simulink model "sen_gyro_lib"  (R2020b)
settings: Solver=FixedStepDiscrete  StartTime=0.0  StopTime=20000  FixedStep=sen.imu_rate  RelTol=1e-3
undefined symbols (not defined in the file or in its folder): DiscIntNeverNeededParam, sen, sen_gyro_dyn_zeta, sen_gyro_lpf_wc
libraries: simulink_extras x2
settings Model: Creator=jsint  LastModifiedBy=jsint

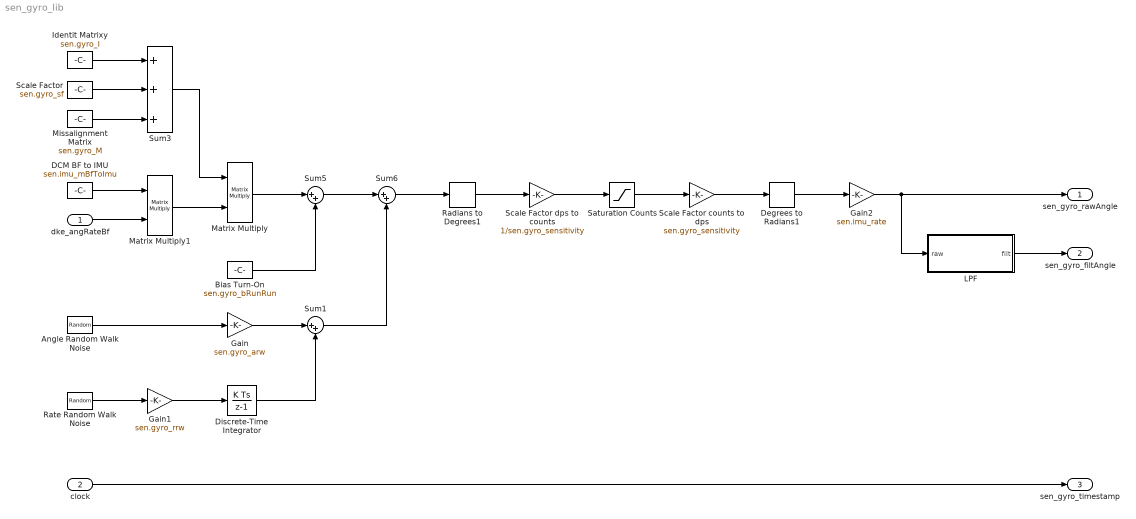
== system sen_gyro_lib ==
  dke_angRateBf : Inport  OutDataTypeStr=double  Unit=rad/s  PortDimensions=[3,1]
  clock : Inport  Port=2  OutDataTypeStr=double  Unit=s  PortDimensions=[1,1]
  Angle Random Walk Noise : RandomNumber  Seed=sen.gyro_arw_seed  SampleTime=sen.imu_rate
  Bias Turn-On : Constant  Value=sen.gyro_bRunRun
  DCM BF to IMU : Constant  Value=sen.imu_mBfToImu
  Degrees to Radians1 : simulink_extras/Transformations/Degrees to Radians
  Discrete-Time Integrator : DiscreteIntegrator  SampleTime=sen.imu_rate  ICPrevOutput=DiscIntNeverNeededParam  ICPrevScaledInput=DiscIntNeverNeededParam
  Gain : Gain  Gain=sen.gyro_arw
  Gain1 : Gain  Gain=sen.gyro_rrw
  Gain2 : Gain  Gain=sen.imu_rate
  Identit Matrixy : Constant  Value=sen.gyro_I
  LPF : Subsystem
  Matrix Multiply : Product  Multiplication=Matrix(*)
  Matrix Multiply1 : Product  Multiplication=Matrix(*)
  Missalignment Matrix : Constant  Value=sen.gyro_M
  Radians to Degrees1 : simulink_extras/Transformations/Radians to Degrees
  Rate Random Walk Noise : RandomNumber  Seed=sen.gyro_rrw_seed  SampleTime=sen.imu_rate
  "Saturation Counts " : Saturate  UpperLimit=2^23  LowerLimit=-2^23
  Scale Factor : Constant  Value=sen.gyro_sf
  "Scale Factor counts to dps " : Gain  Gain=sen.gyro_sensitivity
  "Scale Factor dps to counts " : Gain  Gain=1/sen.gyro_sensitivity
  Sum1 : Sum  Inputs=|++
  Sum3 : Sum  Inputs=+++
  Sum5 : Sum  Inputs=|++
  Sum6 : Sum  Inputs=|++
  sen_gyro_rawAngle : Outport  OutDataTypeStr=double  Unit=rad  PortDimensions=[3,1]
  sen_gyro_filtAngle : Outport  Port=2  OutDataTypeStr=double  Unit=rad  PortDimensions=[3,1]
  sen_gyro_timestamp : Outport  Port=3  OutDataTypeStr=double  Unit=s  PortDimensions=[1,1]
  wires:
  "Scale Factor counts to dps "/1 -> Degrees to Radians1/1
  Gain1/1 -> Discrete-Time Integrator/1
  Missalignment Matrix/1 -> Sum3/3
  Matrix Multiply/1 -> Sum5/1
  Identit Matrixy/1 -> Sum3/1
  Gain/1 -> Sum1/1
  Sum6/1 -> Radians to Degrees1/1
  "Saturation Counts "/1 -> "Scale Factor counts to dps "/1
  Rate Random Walk Noise/1 -> Gain1/1
  Sum1/1 -> Sum6/2
  Discrete-Time Integrator/1 -> Sum1/2
  Degrees to Radians1/1 -> Gain2/1
  Gain2/1 -> sen_gyro_rawAngle/1, LPF/1(raw)
  Angle Random Walk Noise/1 -> Gain/1
  Sum5/1 -> Sum6/1
  "Scale Factor dps to counts "/1 -> "Saturation Counts "/1
  Radians to Degrees1/1 -> "Scale Factor dps to counts "/1
  Scale Factor/1 -> Sum3/2
  Sum3/1 -> Matrix Multiply/1
  Bias Turn-On/1 -> Sum5/2
  LPF/1(filt) -> sen_gyro_filtAngle/1
  clock/1 -> sen_gyro_timestamp/1
  Matrix Multiply1/1 -> Matrix Multiply/2
  dke_angRateBf/1 -> Matrix Multiply1/2
  DCM BF to IMU/1 -> Matrix Multiply1/1

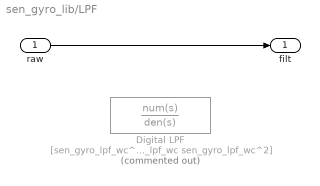
== system sen_gyro_lib/LPF ==
  raw : Inport
  "Digital LPF " : TransferFcn  Commented=on  Numerator=[sen_gyro_lpf_wc^2]  Denominator=[1 2*sen_gyro_dyn_zeta*sen_gyro_lpf_wc sen_gyro_lpf_wc^2]
  filt : Outport
  wires:
  raw/1 -> filt/1
